simulink model "MotorStartup_harness"  (R2024a)
settings: Solver=FixedStepAuto  StartTime=0.0  StopTime=inf  RelTol=1e-3
model workspace (MAT data in the model file):
  mdlWSDbList = "tramontina_database_mobotic.dbc"
undefined symbols (not defined in the file or in its folder): Down, Pull
libraries: speedgoatlib_IO60X_IO69X x2, tramontina_database_moboticlib x2, speedgoatlib_IO691 x1
settings Model: Creator=rodri  LastModifiedBy=rodri
settings SolverCC: ConcurrentTasks=on  PositivePriorityOrder=on
settings OptimizationCC: BlockReduction=off  OptimizeBlockIOStorage=off
settings DebuggingCC: TasksWithSamePriorityMsg=none
settings HardwareCC: ProdBitPerLong=64  ProdLongLongMode=on  ProdHWDeviceType=Intel->x86-64 (Linux 64)
settings SFSimCC: MATLABDynamicMemAlloc=off
settings RTWCC: Description=Speedgoat Real-Time Target Machine  SystemTargetFile=speedgoat.tlc  TemplateMakefile=slrealtime_default_tmf  Toolchain=Simulink Real-Time Toolchain  BuildConfiguration=Faster Runs  CodeExecutionProfiling=on  TargetLang=C++
settings CodeAppCC: MaxIdLength=127
settings SimulinkRealTimeTargetCC: InstructionSetFMA=off  LogToMDFFile=off

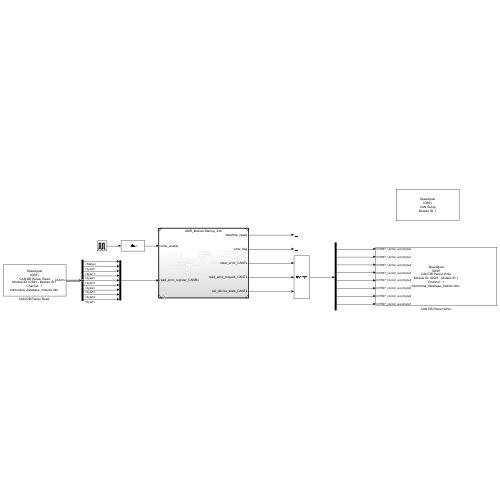
[thumbnail: Simulink's stored preview of the top-level diagram]
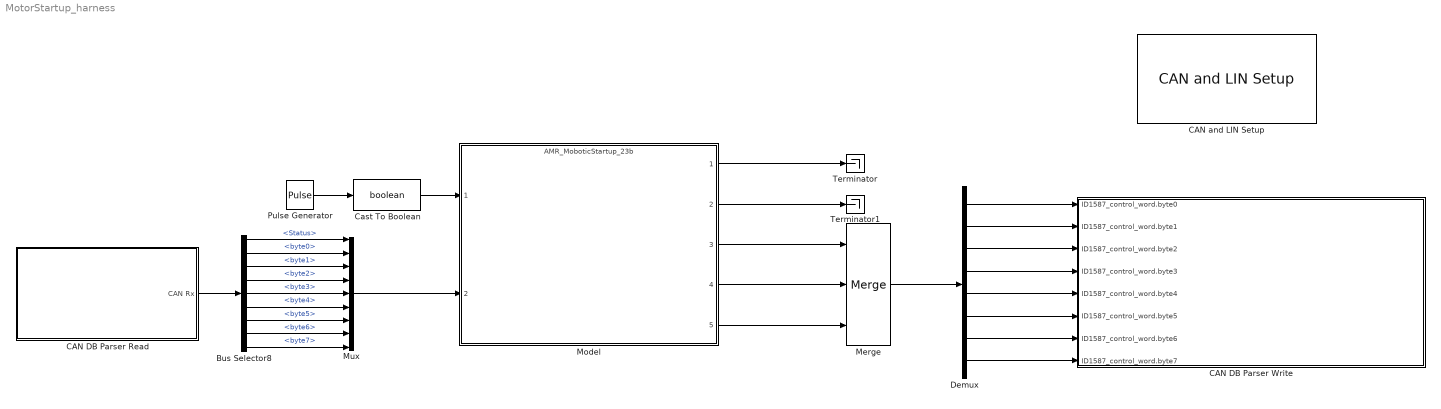
== system MotorStartup_harness ==
  Bus Selector8 : BusSelector  OutputSignals=ID1587_control_word.MessageStatus.Status,ID1587_control_word.byte0,ID1587_control_word.byte1,ID1587_control_word.byte2,ID1587_control_word.byte3,ID1587_control_word.byte4,ID1587_control_word.byte5,ID1587_control_word.byte6,ID1587_control_word.byte7
  "CAN DB Parser Read " : Subsystem
      settings: OpenFcn=sg_can.OpenFcnRead;
      mask Help: eval('sg.utils.help.show(''io_main/refentry_ref_can_ofa_parsing_read'');')
      mask Display: disp('Speedgoat\nIO691\nCAN DB Parser Read\nModule ID: IO691 - Module ID 1\nChannel:  1\ntramontina_database_mobotic.dbc ');
  "CAN DB Parser Write " : Subsystem
      settings: OpenFcn=sg_can.OpenFcnWrite;
      mask Help: eval('sg.utils.help.show(''io_main/refentry_ref_can_ofa_parsing_write'');')
      mask Display: disp('Speedgoat\nIO691\nCAN DB Parser Write\nModule ID: IO691 - Module ID 1\nChannel:  1\ntramontina_database_mobotic.dbc ');
  "CAN and LIN Setup " : speedgoatlib_IO691/CAN and LIN Setup   moduleInitValues="[691    1    1   -1   -1]"  id=1  moduleType=IO691  pciSlot=-1  canChn1=CAN (HS)  canChn2=Disabled  canChn3=Disabled  canChn4=Disabled  linChn1=Disabled  linChn2=Disabled  canInitStructArray=[]  canTermStructArray=[]  gpioChnx=Disabled  canChn1InitValues="[2   2   8   1  16   3  19   2   2   5   2   0]"  arbBdrChn1=500 kBaud  clockDividerChn1=Enable  arbManBdrChn1=[8,1,16,3]  fdBdrChn1=5.0 MBaud  fdManBdrChn1=[2,2,5,2]  termResistor1=off  canChn2InitValues="[1   0   2   8  31   8  19   2   2   5   2   0]"  arbBdrChn2=1.0 MBaud  clockDividerChn2=Enable  arbManBdrChn2=[2,8,31,8]  fdBdrChn2=5.0 MBaud  fdManBdrChn2=[2,2,5,2]  termResistor2=off  canChn3InitValues="[1   0   2   8  31   8  19   2   2   5   2   0]"  arbBdrChn3=1.0 MBaud  clockDividerChn3=Enable  arbManBdrChn3=[2,8,31,8]  fdBdrChn3=5.0 MBaud  fdManBdrChn3=[2,2,5,2]  termResistor3=off  canChn4InitValues="[1   0   2   8  31   8  19   2   2   5   2   0]"  arbBdrChn4=1.0 MBaud  clockDividerChn4=Enable  arbManBdrChn4=[2,8,31,8]  fdBdrChn4=5.0 MBaud  fdManBdrChn4=[2,2,5,2]  termResistor4=off  linChn1InitValues="[0  9600]"  linBtrChn1=9600  linChn2InitValues="[0  9600]"  linBtrChn2=9600  doInitTermStruct="[0  5  0  0  0]"  parDoChannels=[1 2]  parDoVoltage=5  parDoInitValues=0  parDoReset=1  parNumOfDoS=0  parDiChannels=[3 4]  parDiVoltage=5  parDiPull=Pull-Down
      settings: LibrarySourceBlock=speedgoatlib_IO602_IO691/CAN and LIN Setup
  Cast To Boolean : DataTypeConversion  OutDataTypeStr=boolean  SaturateOnIntegerOverflow=off  RndMeth=Floor
  Demux : Demux  Outputs=8
  Merge : Merge  Inputs=3
  Model : ModelReference  ModelNameDialog=AMR_MoboticStartup_23b.slx  SimulationMode=Normal  ModelReferenceVersion=2.17
  Mux : Mux  Inputs=9
  Pulse Generator : DiscretePulseGenerator  PulseType=Time based  Period=10  PulseWidth=5
  Terminator : Terminator
  Terminator1 : Terminator
  wires:
  Pulse Generator/1 -> Cast To Boolean/1
  Cast To Boolean/1 -> Model/1
  Merge/1 -> Demux/1
  Model/4 -> Merge/2
  Model/3 -> Merge/1
  Model/5 -> Merge/3
  Demux/2 -> "CAN DB Parser Write "/2(ID1587_control_word.byte1)
  Demux/1 -> "CAN DB Parser Write "/1(ID1587_control_word.byte0)
  Demux/3 -> "CAN DB Parser Write "/3(ID1587_control_word.byte2)
  Demux/4 -> "CAN DB Parser Write "/4(ID1587_control_word.byte3)
  Demux/5 -> "CAN DB Parser Write "/5(ID1587_control_word.byte4)
  Demux/6 -> "CAN DB Parser Write "/6(ID1587_control_word.byte5)
  Demux/7 -> "CAN DB Parser Write "/7(ID1587_control_word.byte6)
  Demux/8 -> "CAN DB Parser Write "/8(ID1587_control_word.byte7)
  Bus Selector8/4 -> Mux/4  "<byte2>"
  Bus Selector8/9 -> Mux/9  "<byte7>"
  Bus Selector8/5 -> Mux/5  "<byte3>"
  Bus Selector8/8 -> Mux/8  "<byte6>"
  Bus Selector8/2 -> Mux/2  "<byte0>"
  Bus Selector8/3 -> Mux/3  "<byte1>"
  Bus Selector8/7 -> Mux/7  "<byte5>"
  Bus Selector8/6 -> Mux/6  "<byte4>"
  "CAN DB Parser Read "/1(CAN Rx) -> Bus Selector8/1
  Mux/1 -> Model/2
  Bus Selector8/1 -> Mux/1  "<Status>"
  Model/1 -> Terminator/1
  Model/2 -> Terminator1/1

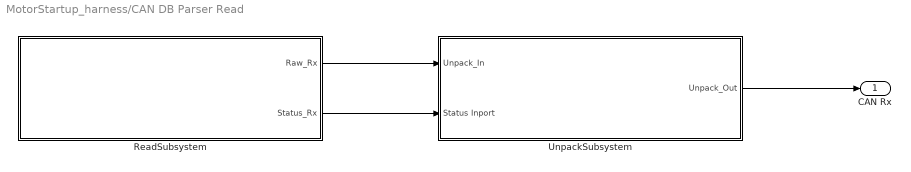
== system MotorStartup_harness/CAN DB Parser Read  ==
  ReadSubsystem : Subsystem
  UnpackSubsystem : Subsystem
  CAN Rx : Outport
  wires:
  ReadSubsystem/1(Raw_Rx) -> UnpackSubsystem/1(Unpack_In)
  ReadSubsystem/2(Status_Rx) -> UnpackSubsystem/2(Status Inport)
  UnpackSubsystem/1(Unpack_Out) -> CAN Rx/1

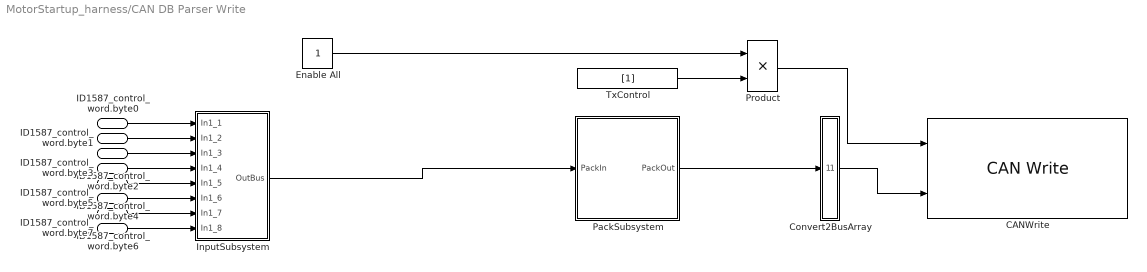
== system MotorStartup_harness/CAN DB Parser Write  ==
  ID1587_control_word.byte0 : Inport
  ID1587_control_word.byte1 : Inport  Port=2
  ID1587_control_word.byte2 : Inport  Port=3
  ID1587_control_word.byte3 : Inport  Port=4
  ID1587_control_word.byte4 : Inport  Port=5
  ID1587_control_word.byte5 : Inport  Port=6
  ID1587_control_word.byte6 : Inport  Port=7
  ID1587_control_word.byte7 : Inport  Port=8
  CANWrite : speedgoatlib_IO60X_IO69X/CAN/CAN Write   moduleType=IO691  id=1  channel=1  canType=CAN (HS)  messageType=CAN (HS)  useBusIn=on  numOfMsg=1  enableInput=on  enableStatusPort=off  ts=-1  initValues=[691 1 -1 0 1 1 0 1 1 1]
  Convert2BusArray : Subsystem
  Enable All : Constant  OutDataTypeStr=boolean
  InputSubsystem : Subsystem
  PackSubsystem : Subsystem
  Product : Product  OutDataTypeStr=uint32
  TxControl : Constant  Value=[1]  OutDataTypeStr=uint32
  wires:
  PackSubsystem/1(PackOut) -> Convert2BusArray/1(InBus)
  Convert2BusArray/1(BusArrayOut) -> CANWrite/2
  Product/1 -> CANWrite/1
  TxControl/1 -> Product/2
  Enable All/1 -> Product/1
  ID1587_control_word.byte0/1 -> InputSubsystem/1(In1_1)
  ID1587_control_word.byte1/1 -> InputSubsystem/2(In1_2)
  ID1587_control_word.byte2/1 -> InputSubsystem/3(In1_3)
  ID1587_control_word.byte3/1 -> InputSubsystem/4(In1_4)
  ID1587_control_word.byte4/1 -> InputSubsystem/5(In1_5)
  ID1587_control_word.byte5/1 -> InputSubsystem/6(In1_6)
  ID1587_control_word.byte6/1 -> InputSubsystem/7(In1_7)
  ID1587_control_word.byte7/1 -> InputSubsystem/8(In1_8)
  InputSubsystem/1(OutBus) -> PackSubsystem/1(PackIn)

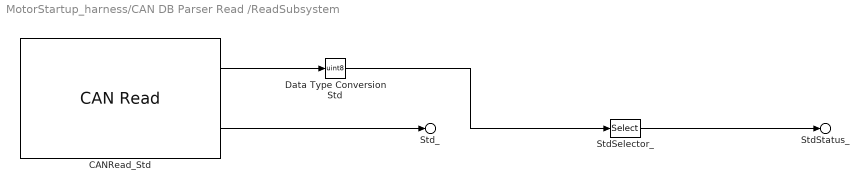
== system MotorStartup_harness/CAN DB Parser Read /ReadSubsystem ==
  CANRead_Std : speedgoatlib_IO60X_IO69X/CAN/CAN Read   moduleType=IO691  id=1  channel=1  canType=CAN (HS)  messageType=CAN (HS)  useBusOut=on  HasMulRead=Specify by IDs  MsgIDlist=[1587]  isEFF=off  LabelInHex=off  enableInput=off  initValues=[691 1 -1 0 1 1 0 1 2 0 1 1587]  ts=-1
  Data Type ConversionStd : DataTypeConversion  OutDataTypeStr=uint8  SaturateOnIntegerOverflow=off  RndMeth=Floor
  StdSelector_ : Selector  IndexOptions=Index vector (dialog)  Indices=1  OutputSizes=1
  Std_ : Outport  PortName=Raw_Rx  Element=Std.ID1587
  StdStatus_ : Outport  Port=2  PortName=Status_Rx  Element=Std.ID1587
  wires:
  CANRead_Std/1 -> Data Type ConversionStd/1
  CANRead_Std/2 -> Std_/1
  Data Type ConversionStd/1 -> StdSelector_/1
  StdSelector_/1 -> StdStatus_/1

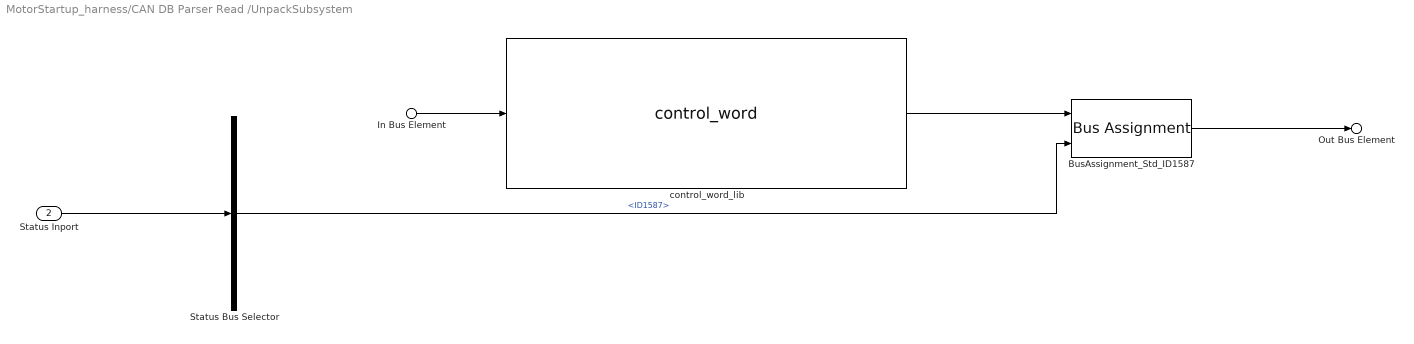
== system MotorStartup_harness/CAN DB Parser Read /UnpackSubsystem ==
  In Bus Element : Inport  PortName=Unpack_In  Element=Std.ID1587
  Status Inport : Inport  Port=2
  BusAssignment_Std_ID1587 : BusAssignment  AssignedSignals=MessageStatus.Status
  Status Bus Selector : BusSelector  OutputSignals=Std.ID1587
  control_word_lib : tramontina_database_moboticlib/CAN unpack/control_word  SystemSampleTime=-1  VariantActivationTime=update diagram  AllowFlexibleInterface=on  Latency=0  AutoFrameSizeCalculation=off
  Out Bus Element : Outport  PortName=Unpack_Out  Element=ID1587_control_word
  wires:
  In Bus Element/1 -> control_word_lib/1
  control_word_lib/1 -> BusAssignment_Std_ID1587/1
  BusAssignment_Std_ID1587/1 -> Out Bus Element/1
  Status Inport/1 -> Status Bus Selector/1
  Status Bus Selector/1 -> BusAssignment_Std_ID1587/2  "<ID1587>"

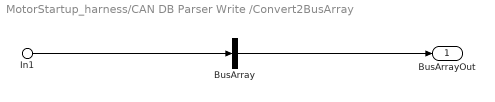
== system MotorStartup_harness/CAN DB Parser Write /Convert2BusArray ==
  In1 : Inport  PortName=InBus  Element=ID1587_control_word
  BusArray : Concatenate  NumInputs=1
  BusArrayOut : Outport
  wires:
  In1/1 -> BusArray/1
  BusArray/1 -> BusArrayOut/1

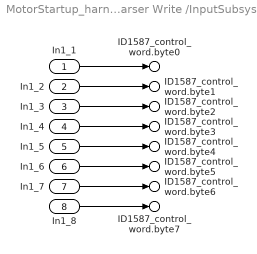
== system MotorStartup_harness/CAN DB Parser Write /InputSubsystem ==
  In1_1 : Inport
  In1_2 : Inport  Port=2
  In1_3 : Inport  Port=3
  In1_4 : Inport  Port=4
  In1_5 : Inport  Port=5
  In1_6 : Inport  Port=6
  In1_7 : Inport  Port=7
  In1_8 : Inport  Port=8
  ID1587_control_word.byte0 : Outport  PortName=OutBus  Element=ID1587_control_word.byte0
  ID1587_control_word.byte1 : Outport  PortName=OutBus  Element=ID1587_control_word.byte1
  ID1587_control_word.byte2 : Outport  PortName=OutBus  Element=ID1587_control_word.byte2
  ID1587_control_word.byte3 : Outport  PortName=OutBus  Element=ID1587_control_word.byte3
  ID1587_control_word.byte4 : Outport  PortName=OutBus  Element=ID1587_control_word.byte4
  ID1587_control_word.byte5 : Outport  PortName=OutBus  Element=ID1587_control_word.byte5
  ID1587_control_word.byte6 : Outport  PortName=OutBus  Element=ID1587_control_word.byte6
  ID1587_control_word.byte7 : Outport  PortName=OutBus  Element=ID1587_control_word.byte7
  wires:
  In1_1/1 -> ID1587_control_word.byte0/1
  In1_2/1 -> ID1587_control_word.byte1/1
  In1_3/1 -> ID1587_control_word.byte2/1
  In1_4/1 -> ID1587_control_word.byte3/1
  In1_5/1 -> ID1587_control_word.byte4/1
  In1_6/1 -> ID1587_control_word.byte5/1
  In1_7/1 -> ID1587_control_word.byte6/1
  In1_8/1 -> ID1587_control_word.byte7/1

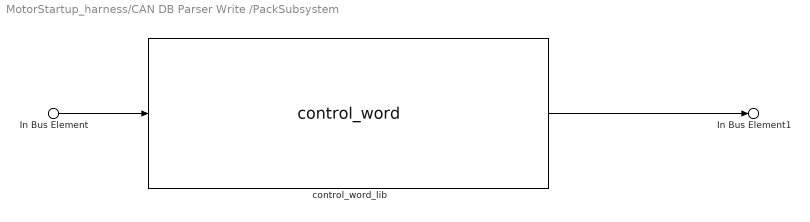
== system MotorStartup_harness/CAN DB Parser Write /PackSubsystem ==
  In Bus Element : Inport  PortName=PackIn  Element=ID1587_control_word
  control_word_lib : tramontina_database_moboticlib/CAN pack/control_word  SystemSampleTime=-1  VariantActivationTime=update diagram  AllowFlexibleInterface=on  Latency=0  AutoFrameSizeCalculation=off
  In Bus Element1 : Outport  PortName=PackOut  Element=ID1587_control_word
  wires:
  In Bus Element/1 -> control_word_lib/1
  control_word_lib/1 -> In Bus Element1/1
